simulink model "chap6_8sim"  (Simulink 7.7)
settings: Solver=ode45  StartTime=0.0  StopTime=10  FixedStep=0.001  RelTol=1e-3
libraries: simulink x1
settings Model: Creator=hp  LastModifiedBy=ljk
settings OptimizationCC: InitFltsAndDblsToZero=on
settings DebuggingCC: SaveWithParameterizedLinksMsg=none  SignalResolutionControl=TryResolveAllWithWarning  SolverPrmCheckMsg=none  MultiTaskDSMMsg=warning  MultiTaskCondExecSysMsg=none  StrictBusMsg=Warning
settings RTWCC: IncludeERTFirstTime=on
settings GRTTargetCC: TargetFcnLib=ansi_tfl_tmw.mat

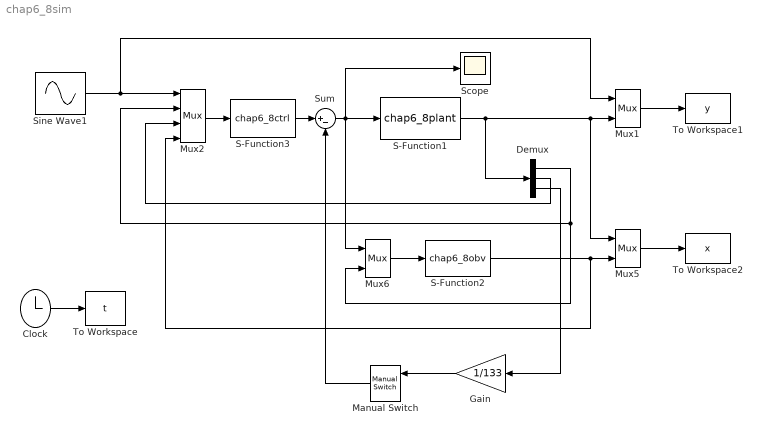
== system chap6_8sim ==
  Clock : Clock
      settings: Decimation=30
  Demux : Demux  Outputs=3
  Gain : Gain  Gain=1/133
  Manual Switch : simulink/Signal Routing/Manual Switch  SystemSampleTime=-1  sw=1  action=0  varsize=off
  Mux1 : Mux  Inputs=2
  Mux2 : Mux
  Mux5 : Mux  Inputs=2
  Mux6 : Mux  Inputs=2
  S-Function1 : S-Function  FunctionName=chap6_8plant  EnableBusSupport=off
  S-Function2 : S-Function  FunctionName=chap6_8obv  EnableBusSupport=off
  S-Function3 : S-Function  FunctionName=chap6_8ctrl  EnableBusSupport=off
  Scope : Scope
  Sine Wave1 : Sin  Frequency=pi  SampleTime=0
  Sum : Sum  Inputs=|+-
  To Workspace : ToWorkspace  VariableName=t  SampleTime=-1  SaveFormat=Array
  To Workspace1 : ToWorkspace  VariableName=y  SampleTime=-1  SaveFormat=Array
  To Workspace2 : ToWorkspace  VariableName=x  SampleTime=-1  SaveFormat=Array
  wires:
  Mux6/1 -> S-Function2/1
  Clock/1 -> To Workspace/1
  S-Function1/1 -> Mux1/2, Mux5/1, Demux/1
  S-Function2/1 -> Mux5/2, Mux2/4
  Mux5/1 -> To Workspace2/1
  Sine Wave1/1 -> Mux1/1, Mux2/1
  Mux1/1 -> To Workspace1/1
  Mux2/1 -> S-Function3/1
  Demux/1 -> Mux6/2, Mux2/2
  S-Function3/1 -> Sum/1
  Sum/1 -> S-Function1/1, Mux6/1, Scope/1
  Demux/2 -> Mux2/3
  Demux/3 -> Gain/1
  Gain/1 -> Manual Switch/1
  Manual Switch/1 -> Sum/2
